simulink library "mweffectlib"  (R2024a)
settings: Solver=VariableStepAuto  StartTime=0.0  StopTime=10.0  RelTol=1e-3
libraries: $bdroot x4
settings Model: Creator=s.maatoug  LastModifiedBy=s.maatoug

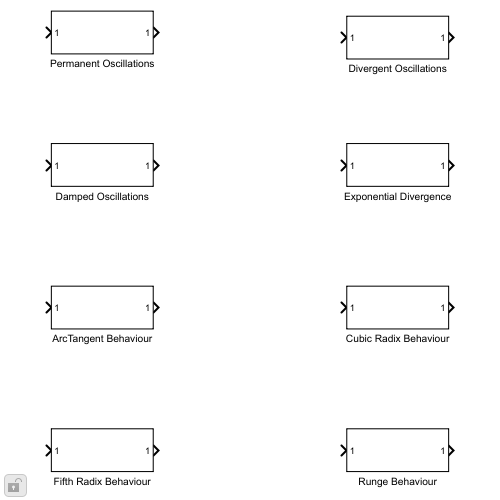
[thumbnail: Simulink's stored preview of the top-level diagram]
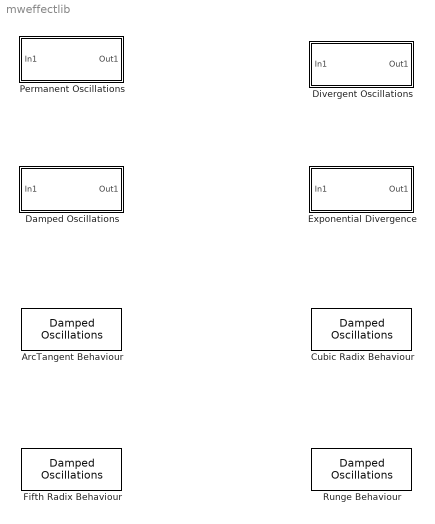
== system mweffectlib ==
  ArcTangent Behaviour : $bdroot/Damped Oscillations  SystemSampleTime=-1  VariantActivationTime=update diagram  AllowFlexibleInterface=on  Latency=0  AutoFrameSizeCalculation=off
  Cubic Radix Behaviour : $bdroot/Damped Oscillations  SystemSampleTime=-1  VariantActivationTime=update diagram  AllowFlexibleInterface=on  Latency=0  AutoFrameSizeCalculation=off
  Damped Oscillations : Subsystem
  Divergent Oscillations : Subsystem
  Exponential Divergence : Subsystem
  Fifth Radix Behaviour : $bdroot/Damped Oscillations  SystemSampleTime=-1  VariantActivationTime=update diagram  AllowFlexibleInterface=on  Latency=0  AutoFrameSizeCalculation=off
  Permanent Oscillations : Subsystem
  Runge Behaviour : $bdroot/Damped Oscillations  SystemSampleTime=-1  VariantActivationTime=update diagram  AllowFlexibleInterface=on  Latency=0  AutoFrameSizeCalculation=off

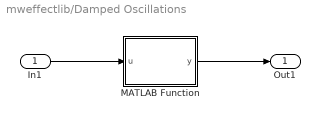
== system mweffectlib/Damped Oscillations ==
  In1 : Inport
  MATLAB Function : MATLAB Function  TreatAsAtomicUnit=on
  Out1 : Outport
  wires:
  In1/1 -> MATLAB Function/1(u)
  MATLAB Function/1(y) -> Out1/1

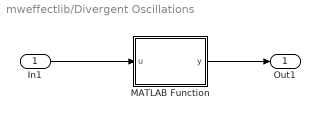
== system mweffectlib/Divergent Oscillations ==
  In1 : Inport
  MATLAB Function : MATLAB Function  TreatAsAtomicUnit=on
  Out1 : Outport
  wires:
  In1/1 -> MATLAB Function/1(u)
  MATLAB Function/1(y) -> Out1/1

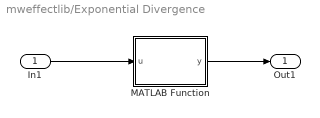
== system mweffectlib/Exponential Divergence ==
  In1 : Inport
  MATLAB Function : MATLAB Function  TreatAsAtomicUnit=on
  Out1 : Outport
  wires:
  In1/1 -> MATLAB Function/1(u)
  MATLAB Function/1(y) -> Out1/1

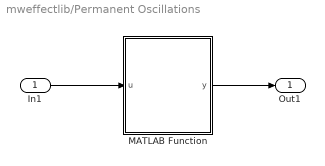
== system mweffectlib/Permanent Oscillations ==
  In1 : Inport
  MATLAB Function : MATLAB Function  StopFcn=|  TreatAsAtomicUnit=on
      | if exist('u_logged', 'var')
      |     propertyCheck = isPermOscillating(u_logged');
      | 
      |     fprintf('Simulazione terminata. Proprietà verificata: %d\n', propertyCheck);
      | end
  Out1 : Outport
  wires:
  In1/1 -> MATLAB Function/1(u)
  MATLAB Function/1(y) -> Out1/1

== matlab function mweffectlib/Permanent Oscillations/MATLAB Function ==
  data: u input; y output
function y = myBlockFunction(u)

    persistent u_values;
    if isempty(u_values)
        u_values = [];
    end

    u_values = [u_values; u]; % save data
    
    assignin('base', 'u_logged', u_values); % Export in workspace

    y = u;
end

== matlab function mweffectlib/Damped Oscillations/MATLAB Function ==
  data: u input; y output
function y = fcn(u)

y = isRunge(u);

end

== matlab function mweffectlib/Exponential Divergence/MATLAB Function ==
  data: u input; y output
function y = fcn(u)

y = isExpDivergent(u);

== matlab function mweffectlib/Divergent Oscillations/MATLAB Function ==
  data: u input; y output
function y = fcn(u)

y = isDivOscillating(u);

end
